simulink model "two_wheeled_mobile_pendulum_system"  (R2018b)
settings: Solver=VariableStepAuto  StartTime=0.0  StopTime=10.0  FixedStep=0.0001  RelTol=1e-3
InitFcn:
  | %%%%%%%%%%%%%%%%%%%%%%%%%
  | %                    SYSTEM PARAMETERS              %
  | %%%%%%%%%%%%%%%%%%%%%%%%%
  | r = 3.15e-2;           % wheel radius
  | mw = 3.15e-2;       % wheel mass
  | l = 8.36e-3;            % distance between COG and wheel axle
  | mb = 0.3604;         % inner body mass
  | d = 0.177;              % wheels distance
  | ja = 8.1367e-5;      % inner body moment of inertia about wheel axle A
  | jb = 5.74620e-4;    % inner body moment of inertia about axis B
  | k = 64;                   % gear ratio
  | jr = 0.12e-7;           % rotor inertia
  | R = 2.3;                  % rotor resistance
  | L = 2.6e-5;             % rotor inductance
  | km = 2.05e-3;        % torque
  | ke = 2.05e-3;         % Back-EMF
  | b = 2.1e-5;             % body-motor viscous friction coefficient
  | fv = 1.8e-4;            % wheels-ground viscous friction coefficient
  | g = 9.81;                % gravity
  | 
  | Tf_aux = [b + fv, 0, -b;
  |           0, b + fv, -b;
  |          -b, -b, 2 * b];
  | 
  | Ta_aux = km * k * [1, 0;
  |                    0, 1;
  |                   -1, -1];
  | 
  | I_aux = ke * k * [1, 0, -1;
  |                   0, 1, -1];
  | 
  | K_aux = ((l^2 * r^2) / d^2) * mb;
libraries: dspindex x3, dspmtrx3 x1
settings Model: Creator=leony  LastModifiedBy=root
settings DebuggingCC: LibraryContextMissingDiagnostic=none
settings SFSimCC: SimUseLocalCustomCode=off
settings RTWCC: RTWUseLocalCustomCode=off

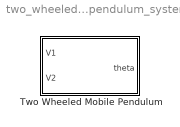
== system two_wheeled_mobile_pendulum_system ==
  Two Wheeled Mobile Pendulum : Subsystem

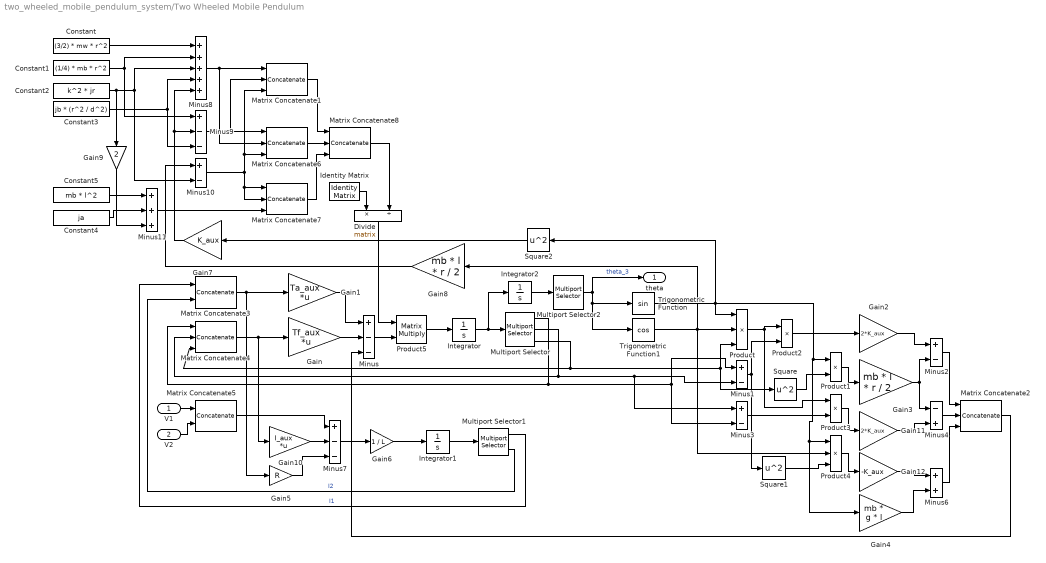
== system two_wheeled_mobile_pendulum_system/Two Wheeled Mobile Pendulum ==
  V1 : Inport
  V2 : Inport  Port=2
  Constant : Constant  Value=(3/2) * mw * r^2
  Constant1 : Constant  Value=(1/4) * mb * r^2
  Constant2 : Constant  Value=k^2 * jr
  Constant3 : Constant  Value=jb * (r^2 / d^2)
  Constant4 : Constant  Value=ja
  Constant5 : Constant  Value=mb * l^2
  Divide : Product  Inputs=*/  Multiplication=Matrix(*)
  Gain : Gain  Gain=Tf_aux  Multiplication=Matrix(K*u)
  Gain1 : Gain  Gain=Ta_aux  Multiplication=Matrix(K*u)
  Gain10 : Gain  Gain=I_aux  Multiplication=Matrix(K*u)
  Gain11 : Gain  Gain=2*K_aux
  Gain12 : Gain  Gain=-K_aux
  Gain2 : Gain  Gain=2*K_aux
  Gain3 : Gain  Gain=mb * l * r / 2
  Gain4 : Gain  Gain=mb * g * l
  Gain5 : Gain  Gain=R
  Gain6 : Gain  Gain=1 / L
  Gain7 : Gain  Gain=K_aux
  Gain8 : Gain  Gain=mb * l * r / 2
  Gain9 : Gain  Gain=2
  Identity Matrix : dspmtrx3/Identity Matrix  Inherit=off  N=3  Ts=1  dataType=double  isSigned=on  wordLen=16  udDataType=sfix(16)  fracBitsMode=Best precision  numFracBits=15  OutDataTypeStr=double  LastOutDataTypeStr=double
      settings: SourceProductName=DSP System Toolbox
  Integrator : Integrator
  Integrator1 : Integrator
  Integrator2 : Integrator
  Matrix Concatenate1 : Concatenate  NumInputs=3  Mode=Multidimensional array  ConcatenateDimension=2
  Matrix Concatenate2 : Concatenate  NumInputs=3  Mode=Multidimensional array
  Matrix Concatenate3 : Concatenate  Mode=Multidimensional array
  Matrix Concatenate4 : Concatenate  NumInputs=3  Mode=Multidimensional array
  Matrix Concatenate5 : Concatenate  Mode=Multidimensional array
  Matrix Concatenate6 : Concatenate  NumInputs=3  Mode=Multidimensional array  ConcatenateDimension=2
  Matrix Concatenate7 : Concatenate  NumInputs=3  Mode=Multidimensional array  ConcatenateDimension=2
  Matrix Concatenate8 : Concatenate  NumInputs=3  Mode=Multidimensional array
  Minus : Sum  Inputs=+--
  Minus{1..3,10} (4 alike) : Sum  Inputs=+-
  Minus11 : Sum  Inputs=+++
  Minus4 : Sum  Inputs=-+
  Minus6 : Sum
  Minus7 : Sum  Inputs=+--
  Minus8 : Sum  Inputs=+++++
  Minus9 : Sum  Inputs=+--
  Multiport Selector : dspindex/Multiport Selector  rowsOrCols=Rows  idxCellArray={1, 2, 3}  idxErrMode=Clip Index
  Multiport Selector1 : dspindex/Multiport Selector  rowsOrCols=Rows  idxCellArray={1, 2}  idxErrMode=Clip Index
  Multiport Selector2 : dspindex/Multiport Selector  rowsOrCols=Rows  idxCellArray={3}  idxErrMode=Clip Index
  Product : Product  Inputs=3
  Product1 : Product
  Product2 : Product
  Product3 : Product
  Product4 : Product  Inputs=3
  Product5 : Product  Multiplication=Matrix(*)
  Square : Math  Operator=square  SaturateOnIntegerOverflow=on
  Square1 : Math  Operator=square  SaturateOnIntegerOverflow=on
  Square2 : Math  Operator=square  SaturateOnIntegerOverflow=on
  Trigonometric Function : Trigonometry
  Trigonometric Function1 : Trigonometry  Operator=cos
  theta : Outport
  wires:
  Minus/1 -> Product5/2
  Product5/1 -> Integrator/1
  Matrix Concatenate8/1 -> Divide/2
  Constant5/1 -> Minus11/1
  Matrix Concatenate7/1 -> Matrix Concatenate8/3
  Multiport Selector1/1 -> Matrix Concatenate3/1  "I1"
  Square2/1 -> Gain7/1
  Matrix Concatenate4/1 -> Gain/1, Gain10/1
  Minus1/1 -> Product2/2, Square1/1
  Matrix Concatenate6/1 -> Matrix Concatenate8/2
  Minus4/1 -> Matrix Concatenate2/2
  Matrix Concatenate5/1 -> Minus7/1
  Gain2/1 -> Minus2/1
  Constant1/1 -> Minus8/2, Minus9/1
  Matrix Concatenate2/1 -> Minus/3
  Integrator2/1 -> Multiport Selector2/1
  Trigonometric Function/1 -> Product4/1, Gain4/1, Product1/1, Product/1, Square2/1
  Product2/1 -> Gain2/1
  Multiport Selector2/1 -> theta/1, Trigonometric Function1/1, Trigonometric Function/1  "theta_3"
  Minus3/1 -> Product3/2
  Trigonometric Function1/1 -> Product/2, Gain8/1, Product4/2
  Constant4/1 -> Minus11/2
  Product1/1 -> Gain3/1
  Minus10/1 -> Matrix Concatenate7/2, Matrix Concatenate7/1, Matrix Concatenate6/3, Matrix Concatenate1/3
  Gain7/1 -> Minus9/2, Minus8/5
  Integrator1/1 -> Multiport Selector1/1
  Divide/1 -> Product5/1
  Minus8/1 -> Matrix Concatenate6/2, Matrix Concatenate1/1
  Gain3/1 -> Minus4/1, Minus2/2
  V1/1 -> Matrix Concatenate5/1
  Multiport Selector/3 -> Square/1, Product/3, Matrix Concatenate4/3
  Gain9/1 -> Minus11/3
  Product/1 -> Product2/1, Product3/1
  Gain4/1 -> Minus6/2
  Minus6/1 -> Matrix Concatenate2/3
  Minus9/1 -> Matrix Concatenate6/1, Matrix Concatenate1/2
  Gain1/1 -> Minus/1
  Gain6/1 -> Integrator1/1
  Product4/1 -> Gain12/1
  Constant/1 -> Minus8/1
  Multiport Selector/1 -> Minus3/2, Minus1/1, Matrix Concatenate4/1
  V2/1 -> Matrix Concatenate5/2
  Identity Matrix/1 -> Divide/1
  Multiport Selector/2 -> Minus1/2, Minus3/1, Matrix Concatenate4/2
  Matrix Concatenate3/1 -> Gain5/1, Gain1/1
  Gain10/1 -> Minus7/2
  Constant3/1 -> Minus8/4, Minus9/3
  Gain12/1 -> Minus6/1
  Square/1 -> Product1/2
  Gain11/1 -> Minus4/2
  Integrator/1 -> Integrator2/1, Multiport Selector/1
  Constant2/1 -> Minus8/3, Minus10/2, Gain9/1
  Square1/1 -> Product4/3
  Minus11/1 -> Matrix Concatenate7/3
  Gain5/1 -> Minus7/3
  Matrix Concatenate1/1 -> Matrix Concatenate8/1
  Gain8/1 -> Minus10/1
  Product3/1 -> Gain11/1
  Gain/1 -> Minus/2
  Minus7/1 -> Gain6/1
  Minus2/1 -> Matrix Concatenate2/1
  Multiport Selector1/2 -> Matrix Concatenate3/2  "I2"
